simulink model "crowther_and_potts"  (R2021b)
settings: Solver=ode14x  StartTime=0.0  StopTime=10.0  FixedStep=1e-3  RelTol=1e-3
values from neighbouring files (symbols this model uses):
  amb = evalin( 'base', 'amb')    [flatball_6dof_eqom.m]
  disc = evalin( 'base', 'disc')    [flatball_6dof_eqom.m]    (also in flatball_6dof_init.m = struct; flatball_init_disc_params.m = struct)
  Y0 = [0 0 -1, 0 15*C.DEG2RAD 0, 15 0 0, 0 0 (2*15*0.29/disc.d)]    [flatball_6dof_eqom.m]
libraries: simulink x1
settings Model: Creator=schae  LastModifiedBy=schae
settings DataIOCC: ReturnWorkspaceOutputsName=simout

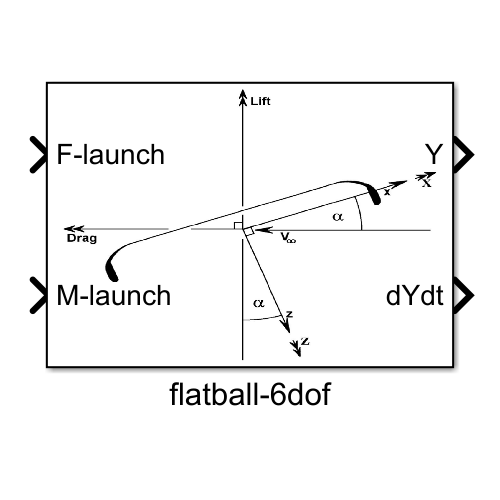
[thumbnail: Simulink's stored preview of the top-level diagram]
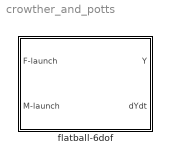
== system crowther_and_potts ==
  flatball-6dof : Subsystem
      mask Display: image('C:\.local\desktop\misc.protolabs\flatball-aero-ssl\arxiv\img\screenshots\flatball-6dof.png'); % Use "Edit Image" on toolstrip to change.

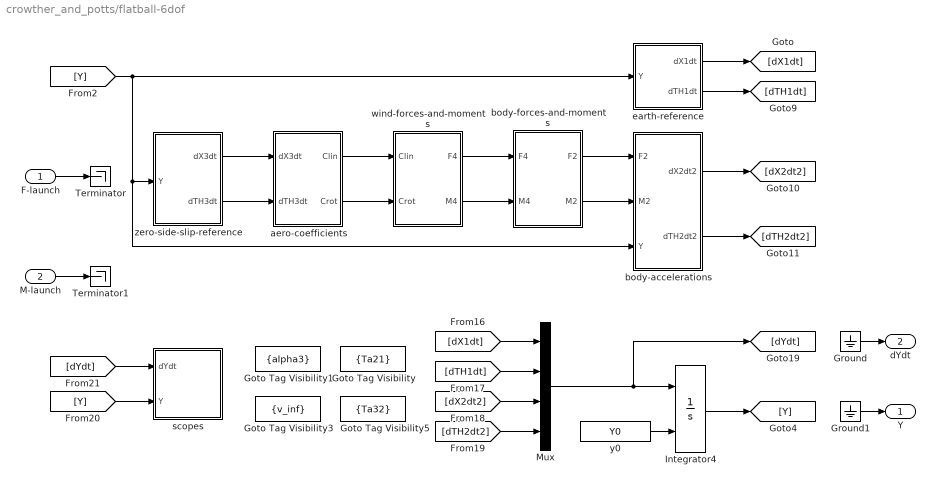
== system crowther_and_potts/flatball-6dof ==
  F-launch : Inport
  M-launch : Inport  Port=2
  Goto Tag Visibility : GotoTagVisibility  GotoTag=Ta21
  Goto Tag Visibility1 : GotoTagVisibility  GotoTag=alpha3
  Goto Tag Visibility3 : GotoTagVisibility  GotoTag=v_inf
  Goto Tag Visibility5 : GotoTagVisibility  GotoTag=Ta32
  Ground : Ground
  Ground1 : Ground
  Integrator4 : Integrator  InitialConditionSource=external
  Mux : Mux
  Terminator : Terminator
  Terminator1 : Terminator
  aero-coefficients : Subsystem
  body-accelerations : Subsystem
  body-forces-and-moments : Subsystem
  earth-reference : Subsystem
  scopes : Subsystem
  wind-forces-and-moments : Subsystem
  y0 : Constant  Value=Y0
  zero-side-slip-reference : Subsystem
  Y : Outport
  dYdt : Outport  Port=2
  wires:
  Ground1/1 -> Y/1
  M-launch/1 -> Terminator1/1
  Ground/1 -> dYdt/1
  wind-forces-and-moments/2(M4) -> body-forces-and-moments/2(M4)
  body-forces-and-moments/2(M2) -> body-accelerations/2(M2)
  wind-forces-and-moments/1(F4) -> body-forces-and-moments/1(F4)
  Mux/1 -> Integrator4/1, [dYdt]
  [dX1dt] -> Mux/1
  aero-coefficients/1(Clin) -> wind-forces-and-moments/1(Clin)
  body-accelerations/1(dX2dt2) -> [dX2dt2]
  [dX2dt2] -> Mux/3
  aero-coefficients/2(Crot) -> wind-forces-and-moments/2(Crot)
  [dTH1dt] -> Mux/2
  [Y] -> scopes/2(Y)
  body-forces-and-moments/1(F2) -> body-accelerations/1(F2)
  zero-side-slip-reference/2(dTH3dt) -> aero-coefficients/2(dTH3dt)
  earth-reference/1(dX1dt) -> [dX1dt]
  earth-reference/2(dTH1dt) -> [dTH1dt]
  body-accelerations/2(dTH2dt2) -> [dTH2dt2]
  [dTH2dt2] -> Mux/4
  F-launch/1 -> Terminator/1
  Integrator4/1 -> [Y]
  [dYdt] -> scopes/1(dYdt)
  zero-side-slip-reference/1(dX3dt) -> aero-coefficients/1(dX3dt)
  [Y] -> earth-reference/1(Y), body-accelerations/3(Y), zero-side-slip-reference/1(Y)
  y0/1 -> Integrator4/2

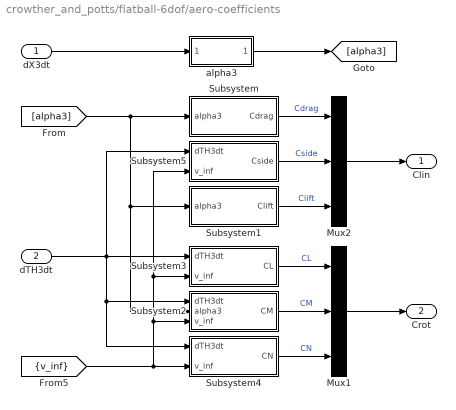
== system crowther_and_potts/flatball-6dof/aero-coefficients ==
  dX3dt : Inport
  dTH3dt : Inport  Port=2
  Mux1 : Mux  Inputs=3
  Mux2 : Mux  Inputs=3
  Subsystem : Subsystem
  Subsystem1 : Subsystem
  Subsystem2 : Subsystem
  Subsystem3 : Subsystem
  Subsystem4 : Subsystem
  Subsystem5 : Subsystem
  alpha3 : Subsystem
  Clin : Outport
  Crot : Outport  Port=2
  wires:
  dX3dt/1 -> alpha3/1(dX3dt)
  Mux2/1 -> Clin/1
  dTH3dt/1 -> Subsystem3/1(dTH3dt), Subsystem2/1(dTH3dt), Subsystem4/1(dTH3dt), Subsystem5/1(dTH3dt)
  Mux1/1 -> Crot/1
  alpha3/1(alpha3) -> [alpha3]
  [alpha3] -> Subsystem/1(alpha3), Subsystem2/2(alpha3), Subsystem1/1(alpha3)
  Subsystem5/1(Cside) -> Mux2/2  "Cside"
  Subsystem/1(Cdrag) -> Mux2/1  "Cdrag"
  Subsystem1/1(Clift) -> Mux2/3  "Clift"
  Subsystem2/1(CM) -> Mux1/2  "CM"
  [v_inf] -> Subsystem5/2(v_inf), Subsystem3/2(v_inf), Subsystem2/3(v_inf), Subsystem4/2(v_inf)
  Subsystem3/1(CL) -> Mux1/1  "CL"
  Subsystem4/1(CN) -> Mux1/3  "CN"

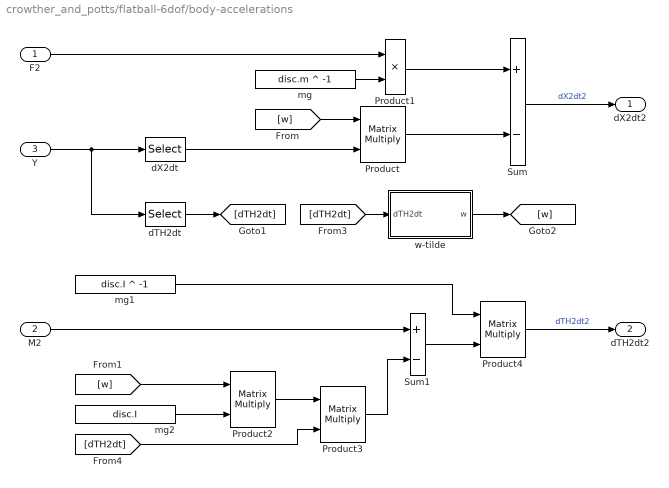
== system crowther_and_potts/flatball-6dof/body-accelerations ==
  F2 : Inport
  M2 : Inport  Port=2
  Y : Inport  Port=3
  Product{,2..4} (4 alike) : Product  Multiplication=Matrix(*)
  Product1 : Product  Inputs=**
  Sum : Sum  Inputs=+-
  Sum1 : Sum  Inputs=+-
  dTH2dt : Selector  InputPortWidth=12  IndexOptions=Index vector (dialog)  Indices=[10 11 12]  OutputSizes=1
  dX2dt : Selector  InputPortWidth=12  IndexOptions=Index vector (dialog)  Indices=[7 8 9]  OutputSizes=1
  mg : Constant  Value=disc.m ^ -1
  mg1 : Constant  Value=disc.I ^ -1
  mg2 : Constant  Value=disc.I
  w-tilde : MATLAB Function  TreatAsAtomicUnit=on
  dX2dt2 : Outport
  dTH2dt2 : Outport  Port=2
  wires:
  Y/1 -> dTH2dt/1, dX2dt/1
  Sum/1 -> dX2dt2/1  "dX2dt2"
  M2/1 -> Sum1/1
  Product4/1 -> dTH2dt2/1  "dTH2dt2"
  dX2dt/1 -> Product/2
  F2/1 -> Product1/1
  mg/1 -> Product1/2
  Product1/1 -> Sum/1
  Product/1 -> Sum/2
  w-tilde/1(w) -> [w]
  [w] -> Product/1
  mg2/1 -> Product2/2
  Product2/1 -> Product3/1
  dTH2dt/1 -> [dTH2dt]
  [dTH2dt] -> w-tilde/1(dTH2dt)
  [dTH2dt] -> Product3/2
  mg1/1 -> Product4/1
  [w] -> Product2/1
  Product3/1 -> Sum1/2
  Sum1/1 -> Product4/2

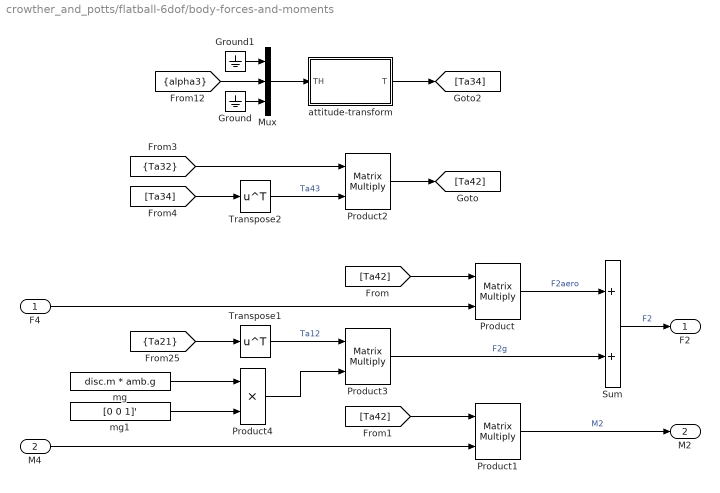
== system crowther_and_potts/flatball-6dof/body-forces-and-moments ==
  F4 : Inport
  M4 : Inport  Port=2
  Ground : Ground
  Ground1 : Ground
  Mux : Mux  Inputs=3
  Product{,1..3} (4 alike) : Product  Multiplication=Matrix(*)
  Product4 : Product
  Sum : Sum  Inputs=2
  Transpose1 : Math  Operator=transpose  SaturateOnIntegerOverflow=on
  Transpose2 : Math  Operator=transpose  SaturateOnIntegerOverflow=on
  attitude-transform : MATLAB Function  TreatAsAtomicUnit=on
  mg : Constant  Value=disc.m * amb.g
  mg1 : Constant  Value=[0 0 1]'
  F2 : Outport
  M2 : Outport  Port=2
  wires:
  [alpha3] -> Mux/2
  F4/1 -> Product/2
  Product/1 -> Sum/1  "F2aero"
  [Ta21] -> Transpose1/1
  Product1/1 -> M2/1  "M2"
  Ground1/1 -> Mux/1
  Mux/1 -> attitude-transform/1(TH)
  Ground/1 -> Mux/3
  attitude-transform/1(T) -> [Ta34]
  [Ta32] -> Product2/1
  [Ta34] -> Transpose2/1
  Product2/1 -> [Ta42]
  [Ta42] -> Product/1
  [Ta42] -> Product1/1
  Sum/1 -> F2/1  "F2"
  Product3/1 -> Sum/2  "F2g"
  Product4/1 -> Product3/2
  Transpose2/1 -> Product2/2  "Ta43"
  mg/1 -> Product4/1
  mg1/1 -> Product4/2
  Transpose1/1 -> Product3/1  "Ta12"
  M4/1 -> Product1/2

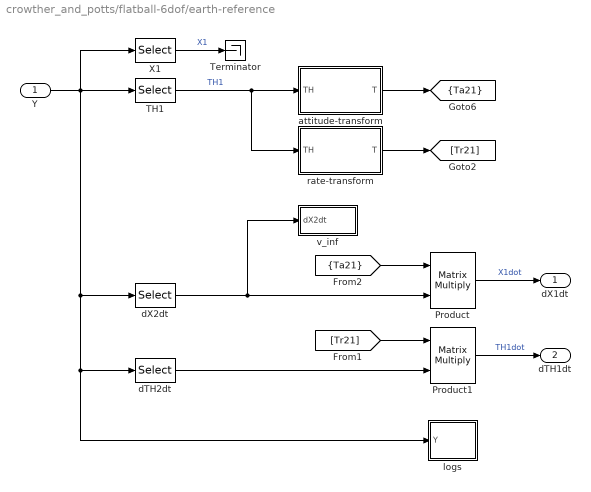
== system crowther_and_potts/flatball-6dof/earth-reference ==
  Y : Inport
  Product : Product  Multiplication=Matrix(*)
  Product1 : Product  Multiplication=Matrix(*)
  TH1 : Selector  InputPortWidth=12  IndexOptions=Index vector (dialog)  Indices=[4 5 6]  OutputSizes=1
  Terminator : Terminator
  X1 : Selector  InputPortWidth=12  IndexOptions=Index vector (dialog)  Indices=[1 2 3]  OutputSizes=1
  attitude-transform : MATLAB Function  TreatAsAtomicUnit=on
  dTH2dt : Selector  InputPortWidth=12  IndexOptions=Index vector (dialog)  Indices=[10 11 12]  OutputSizes=1
  dX2dt : Selector  InputPortWidth=12  IndexOptions=Index vector (dialog)  Indices=[7 8 9]  OutputSizes=1
  logs : Subsystem
  rate-transform : MATLAB Function  TreatAsAtomicUnit=on
  v_inf : Subsystem
  dX1dt : Outport
  dTH1dt : Outport  Port=2
  tag scope: Ta21=scoped
  wires:
  Y/1 -> X1/1, logs/1(Y), dTH2dt/1, dX2dt/1, TH1/1
  dX2dt/1 -> v_inf/1(dX2dt), Product/2
  TH1/1 -> rate-transform/1(TH), attitude-transform/1(TH)  "TH1"
  Product/1 -> dX1dt/1  "X1dot"
  Product1/1 -> dTH1dt/1  "TH1dot"
  X1/1 -> Terminator/1  "X1"
  attitude-transform/1(T) -> [Ta21]
  rate-transform/1(T) -> [Tr21]
  [Ta21] -> Product/1
  [Tr21] -> Product1/1
  dTH2dt/1 -> Product1/2

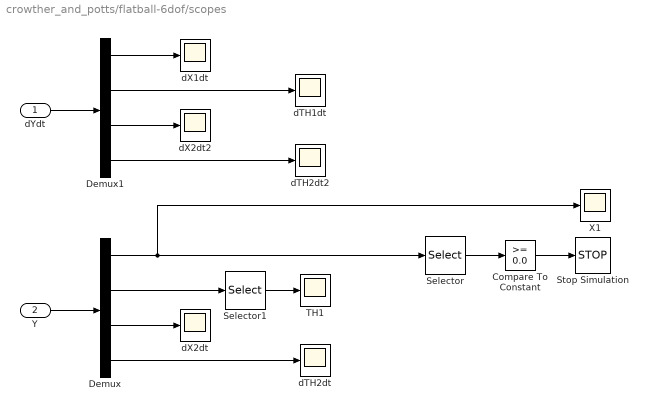
== system crowther_and_potts/flatball-6dof/scopes ==
  dYdt : Inport
  Y : Inport  Port=2
  Compare To Constant : simulink/Logic and Bit Operations/Compare To Constant  relop=>=  const=0.0  OutDataTypeStr=boolean
  Demux : Demux  Outputs=[3 3 3 3]
  Demux1 : Demux  Outputs=[3 3 3 3]
  Selector : Selector  InputPortWidth=3  IndexOptions=Index vector (dialog)  Indices=[3]  OutputSizes=1
  Selector1 : Selector  InputPortWidth=3  IndexOptions=Index vector (dialog)  Indices=[1 2]  OutputSizes=1
  Stop Simulation : Stop
  TH1 : Scope
  X1 : Scope
  dTH1dt : Scope
  dTH2dt : Scope
  dTH2dt2 : Scope
  dX1dt : Scope
  dX2dt : Scope
  dX2dt2 : Scope
  wires:
  Compare To Constant/1 -> Stop Simulation/1
  Selector/1 -> Compare To Constant/1
  Selector1/1 -> TH1/1
  Y/1 -> Demux/1
  Demux/1 -> Selector/1, X1/1
  Demux/2 -> Selector1/1
  Demux/3 -> dX2dt/1
  Demux/4 -> dTH2dt/1
  dYdt/1 -> Demux1/1
  Demux1/1 -> dX1dt/1
  Demux1/2 -> dTH1dt/1
  Demux1/4 -> dTH2dt2/1
  Demux1/3 -> dX2dt2/1

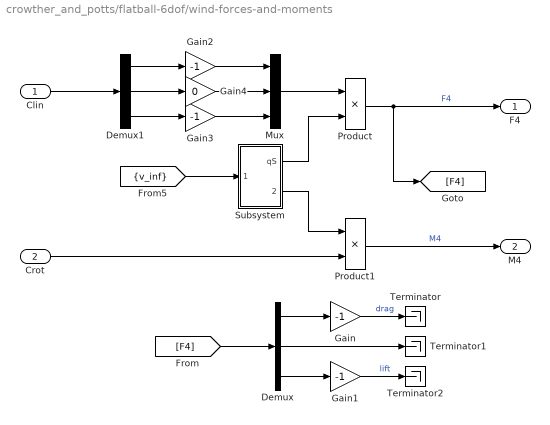
== system crowther_and_potts/flatball-6dof/wind-forces-and-moments ==
  Clin : Inport
  Crot : Inport  Port=2
  Demux : Demux  Outputs=3
  Demux1 : Demux  Outputs=3
  Gain{,1..3} (4 alike) : Gain  Gain=-1
  Gain4 : Gain  Gain=0
  Mux : Mux  Inputs=3
  Product : Product
  Product1 : Product
  Subsystem : Subsystem
  Terminator : Terminator
  Terminator1 : Terminator
  Terminator2 : Terminator
  F4 : Outport
  M4 : Outport  Port=2
  wires:
  Product/1 -> [F4], F4/1  "F4"
  Product1/1 -> M4/1  "M4"
  Demux/2 -> Terminator1/1
  Demux/1 -> Gain/1
  Demux/3 -> Gain1/1
  [F4] -> Demux/1
  Gain1/1 -> Terminator2/1  "lift"
  Gain/1 -> Terminator/1  "drag"
  Demux1/3 -> Gain3/1
  Clin/1 -> Demux1/1
  Demux1/2 -> Gain4/1
  Demux1/1 -> Gain2/1
  Gain3/1 -> Mux/3
  Gain4/1 -> Mux/2
  Gain2/1 -> Mux/1
  Mux/1 -> Product/1
  Subsystem/1(qS) -> Product/2
  Subsystem/2(qSc) -> Product1/1
  Crot/1 -> Product1/2
  [v_inf] -> Subsystem/1(v_inf)

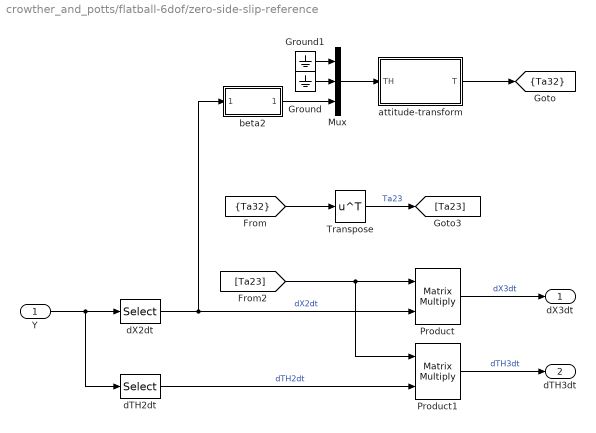
== system crowther_and_potts/flatball-6dof/zero-side-slip-reference ==
  Y : Inport
  Ground : Ground
  Ground1 : Ground
  Mux : Mux  Inputs=3
  Product : Product  Multiplication=Matrix(*)
  Product1 : Product  Multiplication=Matrix(*)
  Transpose : Math  Operator=transpose  SaturateOnIntegerOverflow=on
  attitude-transform : MATLAB Function  TreatAsAtomicUnit=on
  beta2 : Subsystem
  dTH2dt : Selector  InputPortWidth=12  IndexOptions=Index vector (dialog)  Indices=[10 11 12]  OutputSizes=1
  dX2dt : Selector  InputPortWidth=12  IndexOptions=Index vector (dialog)  Indices=[7 8 9]  OutputSizes=1
  dX3dt : Outport
  dTH3dt : Outport  Port=2
  tag scope: Ta32=scoped
  wires:
  Y/1 -> dX2dt/1, dTH2dt/1
  Product1/1 -> dTH3dt/1  "dTH3dt"
  Product/1 -> dX3dt/1  "dX3dt"
  dX2dt/1 -> beta2/1(dX2dt), Product/2  "dX2dt"
  dTH2dt/1 -> Product1/2  "dTH2dt"
  beta2/1(beta2) -> Mux/3
  Mux/1 -> attitude-transform/1(TH)
  Ground/1 -> Mux/2
  Ground1/1 -> Mux/1
  attitude-transform/1(T) -> [Ta32]
  [Ta23] -> Product1/1, Product/1
  [Ta32] -> Transpose/1
  Transpose/1 -> [Ta23]  "Ta23"

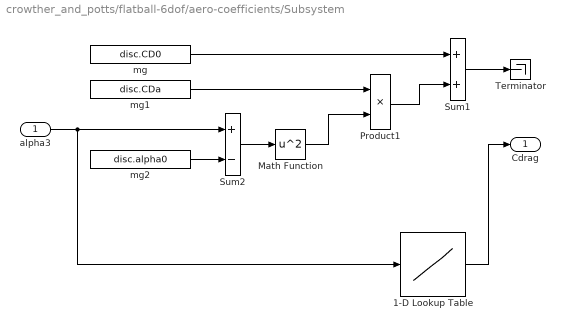
== system crowther_and_potts/flatball-6dof/aero-coefficients/Subsystem ==
  alpha3 : Inport
  1-D Lookup Table : Lookup_n-D  NumberOfTableDimensions=1  BreakpointsForDimension1=disc.aoa_data  Table=disc.Cdrag_data  InterpMethod=Cubic spline  ExtrapMethod=Cubic spline  InternalRulePriority=Speed  RndMeth=Simplest  InputSameDT=on
  Math Function : Math  Operator=square  SaturateOnIntegerOverflow=on
  Product1 : Product  Inputs=**
  Sum1 : Sum
  Sum2 : Sum  Inputs=+-
  Terminator : Terminator
  mg : Constant  Value=disc.CD0
  mg1 : Constant  Value=disc.CDa
  mg2 : Constant  Value=disc.alpha0
  Cdrag : Outport
  wires:
  alpha3/1 -> 1-D Lookup Table/1, Sum2/1
  mg1/1 -> Product1/1
  mg/1 -> Sum1/1
  Product1/1 -> Sum1/2
  Sum2/1 -> Math Function/1
  mg2/1 -> Sum2/2
  Math Function/1 -> Product1/2
  1-D Lookup Table/1 -> Cdrag/1
  Sum1/1 -> Terminator/1

== system crowther_and_potts/flatball-6dof/aero-coefficients/Subsystem1 ==
  alpha3 : Inport
  1-D Lookup Table : Lookup_n-D  NumberOfTableDimensions=1  BreakpointsForDimension1=disc.aoa_data  Table=disc.Clift_data  InterpMethod=Cubic spline  ExtrapMethod=Cubic spline  InternalRulePriority=Speed  RndMeth=Simplest  InputSameDT=on
  Product1 : Product  Inputs=**
  Sum1 : Sum
  Terminator : Terminator
  mg : Constant  Value=disc.CL0
  mg1 : Constant  Value=disc.CLa
  Clift : Outport
  wires:
  Product1/1 -> Sum1/2
  mg/1 -> Sum1/1
  mg1/1 -> Product1/1
  alpha3/1 -> 1-D Lookup Table/1, Product1/2
  1-D Lookup Table/1 -> Clift/1
  Sum1/1 -> Terminator/1

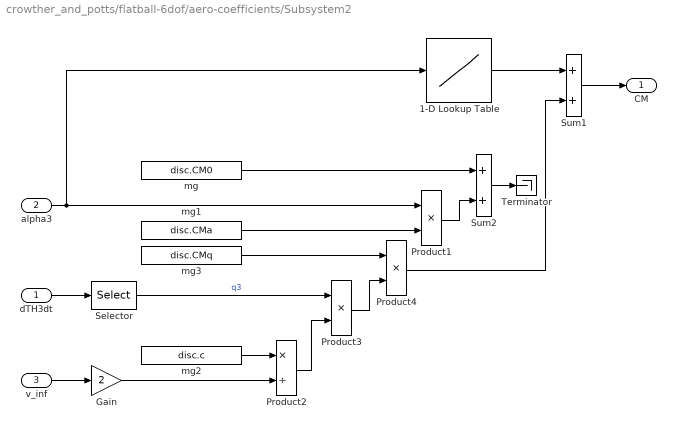
== system crowther_and_potts/flatball-6dof/aero-coefficients/Subsystem2 ==
  dTH3dt : Inport
  alpha3 : Inport  Port=2
  v_inf : Inport  Port=3
  1-D Lookup Table : Lookup_n-D  NumberOfTableDimensions=1  BreakpointsForDimension1=disc.aoa_data  Table=disc.CM_data  InterpMethod=Cubic spline  ExtrapMethod=Cubic spline  InternalRulePriority=Speed  RndMeth=Simplest  InputSameDT=on
  Gain : Gain  Gain=2
  Product1 : Product  Inputs=**
  Product2 : Product  Inputs=*/
  Product3 : Product  Inputs=**
  Product4 : Product  Inputs=**
  Selector : Selector  InputPortWidth=3  IndexOptions=Index vector (dialog)  Indices=[2]  OutputSizes=1
  Sum1 : Sum
  Sum2 : Sum
  Terminator : Terminator
  mg : Constant  Value=disc.CM0
  mg1 : Constant  Value=disc.CMa
  mg2 : Constant  Value=disc.c
  mg3 : Constant  Value=disc.CMq
  CM : Outport
  wires:
  mg2/1 -> Product2/1
  Gain/1 -> Product2/2
  v_inf/1 -> Gain/1
  mg1/1 -> Product1/2
  alpha3/1 -> 1-D Lookup Table/1, Product1/1
  dTH3dt/1 -> Selector/1
  Product2/1 -> Product3/2
  Product3/1 -> Product4/2
  mg3/1 -> Product4/1
  Selector/1 -> Product3/1  "q3"
  Product1/1 -> Sum2/2
  1-D Lookup Table/1 -> Sum1/1
  mg/1 -> Sum2/1
  Sum2/1 -> Terminator/1
  Product4/1 -> Sum1/2
  Sum1/1 -> CM/1

== system crowther_and_potts/flatball-6dof/aero-coefficients/Subsystem3 ==
  dTH3dt : Inport
  v_inf : Inport  Port=2
  Gain : Gain  Gain=2
  Product1 : Product  Inputs=**
  Product2 : Product  Inputs=*/
  Product3 : Product  Inputs=**
  Selector : Selector  InputPortWidth=3  IndexOptions=Index vector (dialog)  Indices=[1]  OutputSizes=1
  mg1 : Constant  Value=disc.CLp
  mg2 : Constant  Value=disc.c
  CL : Outport
  wires:
  Product3/1 -> CL/1
  mg1/1 -> Product1/1
  v_inf/1 -> Gain/1
  mg2/1 -> Product2/1
  dTH3dt/1 -> Selector/1
  Product1/1 -> Product3/1
  Product2/1 -> Product3/2
  Gain/1 -> Product2/2
  Selector/1 -> Product1/2  "p3"

== system crowther_and_potts/flatball-6dof/aero-coefficients/Subsystem4 ==
  dTH3dt : Inport
  v_inf : Inport  Port=2
  Gain : Gain  Gain=2
  Product2 : Product  Inputs=*/
  Product3 : Product  Inputs=**
  Product4 : Product  Inputs=**
  Selector : Selector  InputPortWidth=3  IndexOptions=Index vector (dialog)  Indices=[3]  OutputSizes=1
  mg2 : Constant  Value=disc.c
  mg3 : Constant  Value=disc.CNr
  CN : Outport
  wires:
  mg3/1 -> Product4/1
  Product3/1 -> Product4/2
  Product2/1 -> Product3/2
  dTH3dt/1 -> Selector/1
  v_inf/1 -> Gain/1
  Gain/1 -> Product2/2
  mg2/1 -> Product2/1
  Product4/1 -> CN/1
  Selector/1 -> Product3/1  "r3"

== system crowther_and_potts/flatball-6dof/aero-coefficients/Subsystem5 ==
  dTH3dt : Inport
  v_inf : Inport  Port=2
  Ground : Ground
  Terminator : Terminator
  Terminator1 : Terminator
  Cside : Outport
  wires:
  dTH3dt/1 -> Terminator/1
  Ground/1 -> Cside/1
  v_inf/1 -> Terminator1/1

== system crowther_and_potts/flatball-6dof/aero-coefficients/alpha3 ==
  dX3dt : Inport
  Atan2 : Trigonometry  Operator=atan2
  Selector : Selector  InputPortWidth=3  IndexOptions=Index vector (dialog)  Indices=[3]  OutputSizes=1
  Selector3 : Selector  InputPortWidth=3  IndexOptions=Index vector (dialog)  Indices=[1]  OutputSizes=1
  alpha3 : Outport
  tag scope: alpha3=scoped
  wires:
  dX3dt/1 -> Selector/1, Selector3/1
  Selector3/1 -> Atan2/2  "u3"
  Selector/1 -> Atan2/1  "w3"
  Atan2/1 -> alpha3/1, [alpha3]  "alpha"

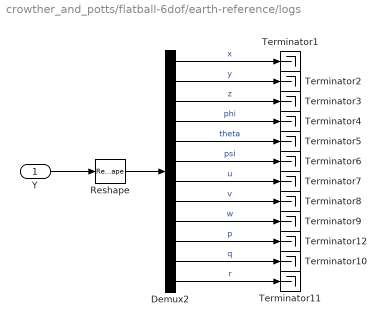
== system crowther_and_potts/flatball-6dof/earth-reference/logs ==
  Y : Inport
  Demux2 : Demux  Outputs=[1 1 1 1 1 1 1 1 1 1 1 1]
  Reshape : Reshape
  Terminator{1..12} (12 alike) : Terminator
  wires:
  Demux2/12 -> Terminator11/1  "r"
  Demux2/5 -> Terminator5/1  "theta"
  Demux2/2 -> Terminator2/1  "y"
  Demux2/4 -> Terminator4/1  "phi"
  Demux2/8 -> Terminator8/1  "v"
  Demux2/11 -> Terminator10/1  "q"
  Reshape/1 -> Demux2/1
  Demux2/10 -> Terminator12/1  "p"
  Demux2/7 -> Terminator7/1  "u"
  Demux2/3 -> Terminator3/1  "z"
  Demux2/1 -> Terminator1/1  "x"
  Y/1 -> Reshape/1
  Demux2/6 -> Terminator6/1  "psi"
  Demux2/9 -> Terminator9/1  "w"

== system crowther_and_potts/flatball-6dof/earth-reference/v_inf ==
  dX2dt : Inport
  Sqrt : Sqrt  SaturateOnIntegerOverflow=on
  Square3 : Math  Operator=square  SaturateOnIntegerOverflow=on
  Sum1 : Sum  Inputs=1
  tag scope: v_inf=scoped
  wires:
  Sqrt/1 -> [v_inf]  "v_inf"
  dX2dt/1 -> Square3/1
  Square3/1 -> Sum1/1
  Sum1/1 -> Sqrt/1

== system crowther_and_potts/flatball-6dof/wind-forces-and-moments/Subsystem ==
  v_inf : Inport
  Gain2 : Gain  Gain=0.5
  Math Function : Math  Operator=square  SaturateOnIntegerOverflow=on
  Product : Product
  Product1 : Product
  Product2 : Product
  S : Constant  Value=disc.S
  c : Constant  Value=disc.c
  rho : Constant  Value=amb.rho
  qS : Outport
  qSc : Outport  Port=2
  wires:
  rho/1 -> Gain2/1
  Gain2/1 -> Product/2
  Math Function/1 -> Product/1
  v_inf/1 -> Math Function/1
  Product/1 -> Product1/1  "q_inf"
  Product1/1 -> Product2/1, qS/1
  Product2/1 -> qSc/1
  c/1 -> Product2/2
  S/1 -> Product1/2

== system crowther_and_potts/flatball-6dof/zero-side-slip-reference/beta2 ==
  dX2dt : Inport
  Atan2 : Trigonometry  Operator=atan2
  Goto3 : Goto  Commented=on  GotoTag=beta2  TagVisibility=scoped
  Selector : Selector  InputPortWidth=3  IndexOptions=Index vector (dialog)  Indices=[2]  OutputSizes=1
  Selector3 : Selector  InputPortWidth=3  IndexOptions=Index vector (dialog)  Indices=[1]  OutputSizes=1
  beta2 : Outport
  wires:
  dX2dt/1 -> Selector/1, Selector3/1
  Selector3/1 -> Atan2/2  "u2"
  Selector/1 -> Atan2/1  "v2"
  Atan2/1 -> beta2/1, Goto3/1  "beta"

== matlab function crowther_and_potts/flatball-6dof/earth-reference/attitude-transform ==
  data: T output; TH input
function T = Ta( TH)
% attitude transformation per Etkin and Reid 1995
phi = TH(1); theta = TH(2); psi = TH(3);
T = [
    cos(theta)*cos(psi), sin(phi)*sin(theta)*cos(psi) - cos(phi)*sin(psi), cos(phi)*sin(theta)*cos(psi) + sin(phi)*sin(psi);
    cos(theta)*sin(psi), sin(phi)*sin(theta)*sin(psi) + cos(phi)*cos(psi), cos(phi)*sin(theta)*sin(psi) - sin(phi)*cos(psi);
    -sin(theta), sin(phi)*cos(theta), cos(phi)*cos(theta)
    ];

== matlab function crowther_and_potts/flatball-6dof/body-accelerations/w-tilde ==
  data: w output; dTH2dt input
function w = w_tilde( dTH2dt)
    p = dTH2dt(1); q = dTH2dt( 2); r = dTH2dt(3);
    w = [0 -r q; r 0 -p; -q p 0];

== matlab function crowther_and_potts/flatball-6dof/zero-side-slip-reference/attitude-transform ==
  data: T output; TH input
function T = Ta( TH)
% attitude transformation per Etkin and Reid 1995
phi = TH(1); theta = TH(2); psi = TH(3);
T = [
    cos(theta)*cos(psi), sin(phi)*sin(theta)*cos(psi) - cos(phi)*sin(psi), cos(phi)*sin(theta)*cos(psi) + sin(phi)*sin(psi);
    cos(theta)*sin(psi), sin(phi)*sin(theta)*sin(psi) + cos(phi)*cos(psi), cos(phi)*sin(theta)*sin(psi) - sin(phi)*cos(psi);
    -sin(theta), sin(phi)*cos(theta), cos(phi)*cos(theta)
    ];

== matlab function crowther_and_potts/flatball-6dof/body-forces-and-moments/attitude-transform ==
  data: T output; TH input
function T = Ta( TH)
% attitude transformation per Etkin and Reid 1995
phi = TH(1); theta = TH(2); psi = TH(3);
T = [
    cos(theta)*cos(psi), sin(phi)*sin(theta)*cos(psi) - cos(phi)*sin(psi), cos(phi)*sin(theta)*cos(psi) + sin(phi)*sin(psi);
    cos(theta)*sin(psi), sin(phi)*sin(theta)*sin(psi) + cos(phi)*cos(psi), cos(phi)*sin(theta)*sin(psi) - sin(phi)*cos(psi);
    -sin(theta), sin(phi)*cos(theta), cos(phi)*cos(theta)
    ];

== matlab function crowther_and_potts/flatball-6dof/earth-reference/rate-transform ==
  data: T output; TH input
function T = Tr( TH)
% euler angle rate transformation per Etkin and Reid 1995
phi = TH(1); theta = TH(2); % psi = TH(3);
T = [
    1, sin(phi)*tan(theta), cos(phi)*tan(theta);
    0, cos(phi), -sin(phi);
    0, sin(phi)*sec(theta), cos(phi)*sec(theta)
    ];
